simulink model "non_linear_feedback"  (R2019a)
settings: Solver=VariableStepAuto  StartTime=0.0  StopTime=10  RelTol=1e-3
settings Model: Creator=iyengar  LastModifiedBy=iyengar

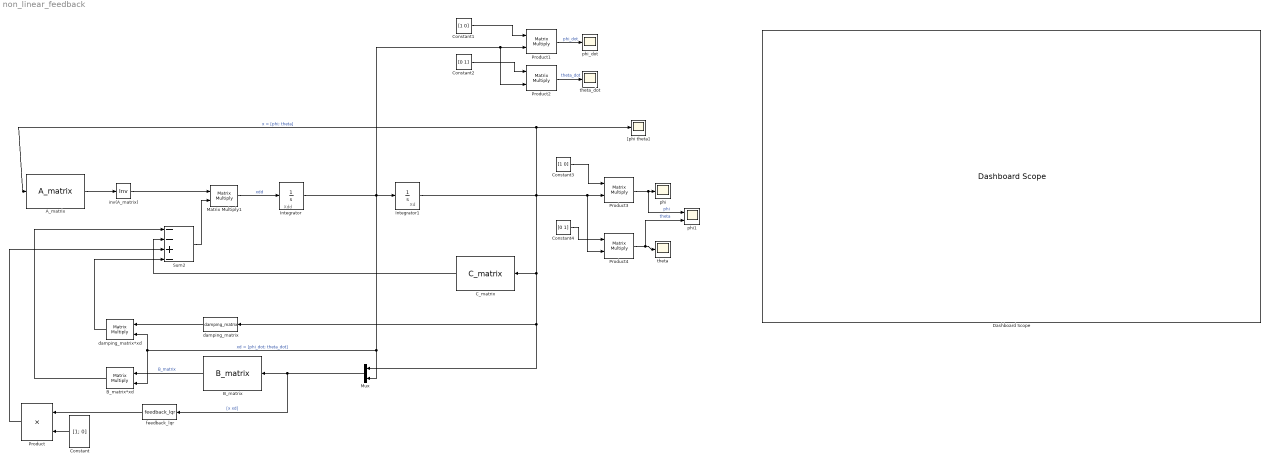
== system non_linear_feedback ==
  note: Xdd
  note: Xd
  "A_matrix " : MATLABFcn  Description=matrix A. 2x2  MATLABFcn=A_matrix  Output1D=off
  B_matrix : MATLABFcn  MATLABFcn=B_matrix  Output1D=off
  B_matrix*xd : Product  Multiplication=Matrix(*)
  C_matrix : MATLABFcn  MATLABFcn=C_matrix  Output1D=off
  Constant : Constant  Value=[1; 0]  VectorParams1D=off
  Constant1 : Constant  Value=[1 0]  VectorParams1D=off
  Constant2 : Constant  Value=[0 1]  VectorParams1D=off
  Constant3 : Constant  Value=[1 0]  VectorParams1D=off
  Constant4 : Constant  Value=[0 1]  VectorParams1D=off
  Dashboard Scope : DashboardScope
  Integrator : Integrator  InitialCondition=[0; 0]
  Integrator1 : Integrator  InitialCondition=[0; 0.01]
  Matrix Multiply1 : Product  Multiplication=Matrix(*)
  Mux : Mux  Inputs=2
  Product : Product
  Product{1..4} (4 alike) : Product  Multiplication=Matrix(*)
  Sum2 : Sum  Inputs=--+-
  "[phi theta]" : Scope
  damping_matrix : MATLABFcn  MATLABFcn=damping_matrix  Output1D=off
  "damping_matrix*xd " : Product  Multiplication=Matrix(*)
  feedback_lqr : MATLABFcn  MATLABFcn=feedback_lqr  Output1D=off
  inv(A_matrix) : Product  Inputs=/  Multiplication=Matrix(*)
  phi : Scope
  phi1 : Scope  NumInputPorts=2
  phi_dot : Scope
  theta : Scope
  theta_dot : Scope
  wires:
  Product2/1 -> theta_dot/1  "theta_dot"
  B_matrix/1 -> B_matrix*xd/1  "B_matrix"
  Constant2/1 -> Product2/1
  Matrix Multiply1/1 -> Integrator/1  "xdd"
  Constant1/1 -> Product1/1
  Product/1 -> Sum2/3
  Product4/1 -> phi1/2, theta/1  "theta"
  inv(A_matrix)/1 -> Matrix Multiply1/1
  Constant/1 -> Product/2
  Mux/1 -> feedback_lqr/1, B_matrix/1  "[x xd]"
  damping_matrix/1 -> "damping_matrix*xd "/1
  Product1/1 -> phi_dot/1  "phi_dot"
  Constant3/1 -> Product3/1
  Integrator/1 -> Product2/2, Product1/2, Integrator1/1, Mux/2, "damping_matrix*xd "/2, B_matrix*xd/2  "xd = [phi_dot; theta_dot]"
  "A_matrix "/1 -> inv(A_matrix)/1
  B_matrix*xd/1 -> Sum2/1
  Integrator1/1 -> "A_matrix "/1, "[phi theta]"/1, Product4/2, Product3/2, damping_matrix/1, Mux/1, C_matrix/1  "x = [phi; theta]"
  Constant4/1 -> Product4/1
  Sum2/1 -> Matrix Multiply1/2
  Product3/1 -> phi1/1, phi/1  "phi"
  C_matrix/1 -> Sum2/2
  feedback_lqr/1 -> Product/1
  "damping_matrix*xd "/1 -> Sum2/4
